simulink model "Example_12_3_1"  (R2018a)
settings: Solver=FixedStepAuto  StartTime=0.0  StopTime=2  FixedStep=0.001  RelTol=1e-3
settings Model: Creator=ahmed  LastModifiedBy=ahmed
settings SolverCC: ShapePreserveControl=EnableAll

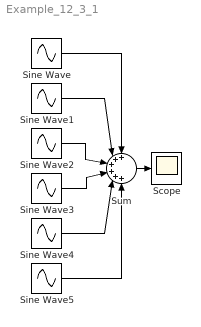
== system Example_12_3_1 ==
  Scope : Scope
  Sine Wave : Sin  Frequency=1*2*pi  SampleTime=0
  Sine Wave1 : Sin  Amplitude=1/3  Frequency=3*2*pi  SampleTime=0
  Sine Wave2 : Sin  Amplitude=1/5  Frequency=5*2*pi  SampleTime=0
  Sine Wave3 : Sin  Amplitude=1/7  Frequency=7*2*pi  SampleTime=0
  Sine Wave4 : Sin  Amplitude=1/9  Frequency=9*2*pi  SampleTime=0
  Sine Wave5 : Sin  Amplitude=1/11  Frequency=11*2*pi  SampleTime=0
  Sum : Sum  Inputs=6
  wires:
  Sum/1 -> Scope/1
  Sine Wave/1 -> Sum/1
  Sine Wave1/1 -> Sum/2
  Sine Wave2/1 -> Sum/3
  Sine Wave3/1 -> Sum/4
  Sine Wave4/1 -> Sum/5
  Sine Wave5/1 -> Sum/6
